simulink model "simulink_test"  (R2023b)
settings: Solver=VariableStepAuto  StartTime=0.0  StopTime=10.0  RelTol=1e-3
values from neighbouring files (symbols this model uses):
  q_test = 1    [class_test2D.m]    (also in class_test3D.m = 1*[1; -1; 0.2]; class_test_rigid.m)
  r2 = BodyTreeOld(J2, B2, 1e-4*ones(n*N_B, 1), 1e-4*ones(n*N_B, 1), 1e-4*ones(n*N_B, 1), 1e-4*ones(n*N_B, 1))    [class_test_rigid.m]    (also in methods_test.m = BodyTree({j2}, {b2}, 1e-4*ones(n, 1), 1e-4*ones(n, 1), 1e-4*)
libraries: SoftRobotics x2
settings Model: Creator=pietro  LastModifiedBy=pietro

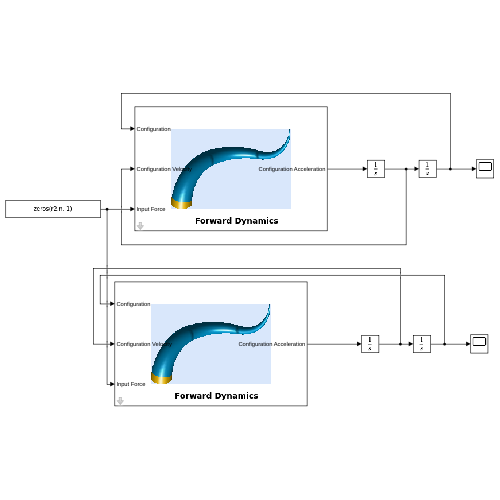
[thumbnail: Simulink's stored preview of the top-level diagram]
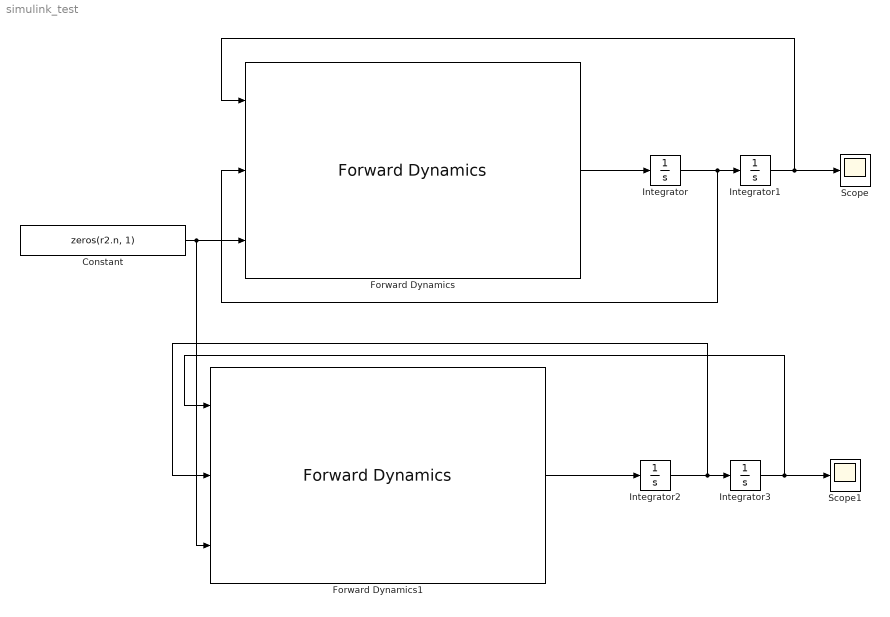
== system simulink_test ==
  Constant : Constant  Value=zeros(r2.n, 1)
  Forward Dynamics : SoftRobotics/Forward Dynamics  RobotModel=r2  SimulateUsing=Code generation
      settings: SourceProductName=Soft Robotics Toolbox
  Forward Dynamics1 : SoftRobotics/Forward Dynamics  RobotModel=r1  SimulateUsing=Code generation
      settings: SourceProductName=Soft Robotics Toolbox
  Integrator : Integrator
  Integrator1 : Integrator  InitialCondition=q_test
  Integrator2 : Integrator
  Integrator3 : Integrator  InitialCondition=q_test
  Scope : Scope
  Scope1 : Scope
  wires:
  Forward Dynamics/1 -> Integrator/1
  Integrator/1 -> Forward Dynamics/2, Integrator1/1
  Integrator1/1 -> Scope/1, Forward Dynamics/1
  Constant/1 -> Forward Dynamics1/3, Forward Dynamics/3
  Forward Dynamics1/1 -> Integrator2/1
  Integrator3/1 -> Scope1/1, Forward Dynamics1/1
  Integrator2/1 -> Forward Dynamics1/2, Integrator3/1
